simulink model "lin_model"  (R2014a)
settings: Solver=ode45  StartTime=0.0  StopTime=0.01  RelTol=1e-3
model workspace (MAT data in the model file):
  Ki = 12447149.4811
  Kd = -86.1936978403
  Kp = 336087.390249
settings Model: Creator=Deadok  LastModifiedBy=Mihail
settings DataIOCC: SignalLoggingSaveFormat=ModelDataLogs
settings OptimizationCC: ExpressionDepthLimit=2147483647
settings DebuggingCC: AlgebraicLoopMsg=none  UnderspecifiedInitializationDetection=Classic  SolverPrmCheckMsg=none  FcnCallInpInsideContextMsg=UseLocalSettings  UnconnectedInputMsg=none  UnconnectedOutputMsg=none  UnconnectedLineMsg=none  StateNameClashWarn=warning
settings GRTTargetCC: CombineOutputUpdateFcns=off  GRTInterface=on

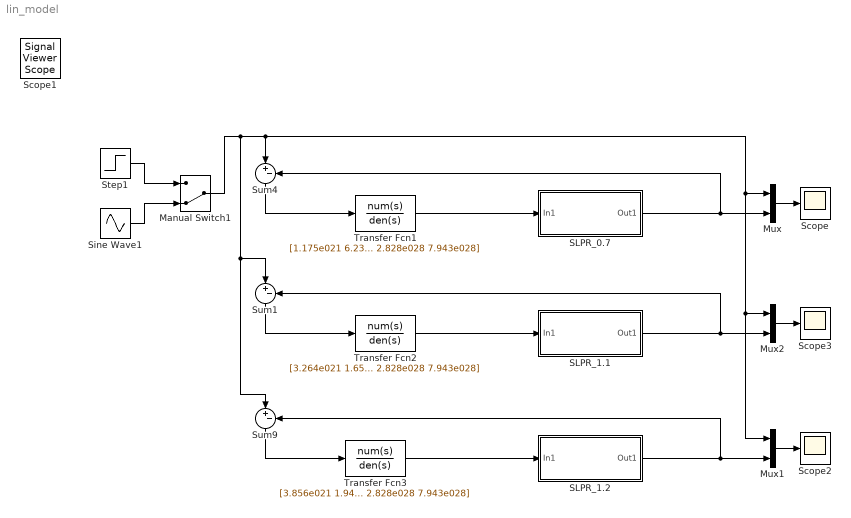
== system lin_model ==
  Manual Switch1 : ManualSwitch  CurrentSetting=0
  Mux : Mux  Inputs=2
  Mux1 : Mux  Inputs=2
  Mux2 : Mux  Inputs=2
  SLPR_0.7 : Subsystem
  SLPR_1.1 : Subsystem
  SLPR_1.2 : Subsystem
  Scope : Scope
      settings: TimeRange=16  YMin=1.832061068702288  YMax=5.832061068702288
  Scope2 : Scope
      settings: TimeRange=16  YMin=1.832061068702288  YMax=5.832061068702288
  Scope3 : Scope
      settings: TimeRange=16  YMin=1.832061068702288  YMax=5.832061068702288  SaveName=ScopeData2
  Sine Wave1 : Sin  Frequency=2000  SampleTime=0
  Step1 : Step  Time=0  SampleTime=0
  Sum1 : Sum  Inputs=|+-
  Sum4 : Sum  Inputs=|+-
  Sum9 : Sum  Inputs=|+-
  Transfer Fcn1 : TransferFcn  Numerator=[1.175e021 6.235e024 6.654e027 1.224e031 2.049e033 4.008e034 4.923e036 2.383e036]  Denominator=[1 1.539e006 8.565e011 2.152e017 2.439e022 1.001e027 2.828e028 7.943e028]
  Transfer Fcn2 : TransferFcn  Numerator=[3.264e021 1.656e025 1.052e028 1.263e031 2.055e033 4.055e034 4.923e036 2.383e036]  Denominator=[1 1.539e006 8.565e011 2.152e017 2.439e022 1.001e027 2.828e028 7.943e028]
  Transfer Fcn3 : TransferFcn  Numerator=[3.856e021 1.946e025 1.147e028 1.272e031 2.057e033 4.065e034 4.923e036 2.383e036]  Denominator=[1 1.539e006 8.565e011 2.152e017 2.439e022 1.001e027 2.828e028 7.943e028]
  Scope1 : SignalViewerScope  IOType=viewer  RefreshTime=0.035000
  wires:
  SLPR_0.7/1(Out1) -> Mux/2, Sum4/2
  Mux/1 -> Scope/1
  SLPR_1.2/1(Out1) -> Mux1/2, Sum9/2
  Sum9/1 -> Transfer Fcn3/1
  Mux1/1 -> Scope2/1
  SLPR_1.1/1(Out1) -> Sum1/2, Mux2/2
  Sine Wave1/1 -> Manual Switch1/2
  Step1/1 -> Manual Switch1/1
  Sum1/1 -> Transfer Fcn2/1
  Mux2/1 -> Scope3/1
  Manual Switch1/1 -> Sum1/1, Sum9/1, Sum4/1, Mux/1, Mux2/1, Mux1/1
  Sum4/1 -> Transfer Fcn1/1
  Transfer Fcn1/1 -> SLPR_0.7/1(In1)
  Transfer Fcn3/1 -> SLPR_1.2/1(In1)
  Transfer Fcn2/1 -> SLPR_1.1/1(In1)

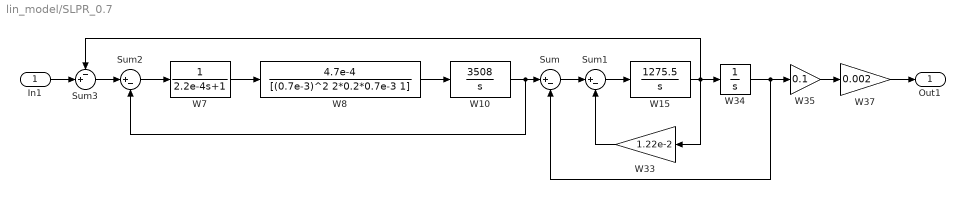
== system lin_model/SLPR_0.7 ==
  In1 : Inport
  Sum : Sum  Inputs=|+-
  Sum1 : Sum  Inputs=|+-
  Sum2 : Sum  Inputs=|+-
  Sum3 : Sum  Inputs=-+|
  W10 : TransferFcn  Numerator=[3508]  Denominator=[1 0]
  W15 : TransferFcn  Numerator=[1275.5]  Denominator=[1 0]
  W33 : Gain  Gain=1.22e-2
  W34 : Integrator
  W35 : Gain  Gain=0.1
  W37 : Gain  Gain=0.002
  W7 : TransferFcn  Denominator=[2.2e-4 1]
  W8 : TransferFcn  Numerator=[4.7e-4]  Denominator=[(0.7e-3)^2 2*0.2*0.7e-3 1]
  Out1 : Outport
  wires:
  W7/1 -> W8/1
  W8/1 -> W10/1
  W10/1 -> Sum2/2, Sum/1
  Sum/1 -> Sum1/1
  Sum1/1 -> W15/1
  W34/1 -> Sum/2, W35/1
  W33/1 -> Sum1/2
  Sum2/1 -> W7/1
  Sum3/1 -> Sum2/1
  W35/1 -> W37/1
  In1/1 -> Sum3/2
  W37/1 -> Out1/1
  W15/1 -> Sum3/1, W33/1, W34/1

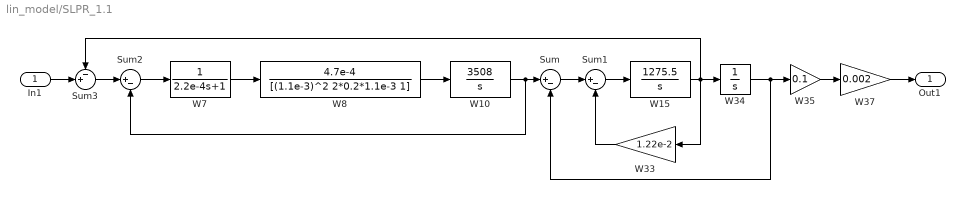
== system lin_model/SLPR_1.1 ==
  In1 : Inport
  Sum : Sum  Inputs=|+-
  Sum1 : Sum  Inputs=|+-
  Sum2 : Sum  Inputs=|+-
  Sum3 : Sum  Inputs=-+|
  W10 : TransferFcn  Numerator=[3508]  Denominator=[1 0]
  W15 : TransferFcn  Numerator=[1275.5]  Denominator=[1 0]
  W33 : Gain  Gain=1.22e-2
  W34 : Integrator
  W35 : Gain  Gain=0.1
  W37 : Gain  Gain=0.002
  W7 : TransferFcn  Denominator=[2.2e-4 1]
  W8 : TransferFcn  Numerator=[4.7e-4]  Denominator=[(1.1e-3)^2 2*0.2*1.1e-3 1]
  Out1 : Outport
  wires:
  W7/1 -> W8/1
  W8/1 -> W10/1
  W10/1 -> Sum2/2, Sum/1
  Sum/1 -> Sum1/1
  Sum1/1 -> W15/1
  W34/1 -> Sum/2, W35/1
  W33/1 -> Sum1/2
  Sum2/1 -> W7/1
  Sum3/1 -> Sum2/1
  W35/1 -> W37/1
  In1/1 -> Sum3/2
  W37/1 -> Out1/1
  W15/1 -> Sum3/1, W33/1, W34/1

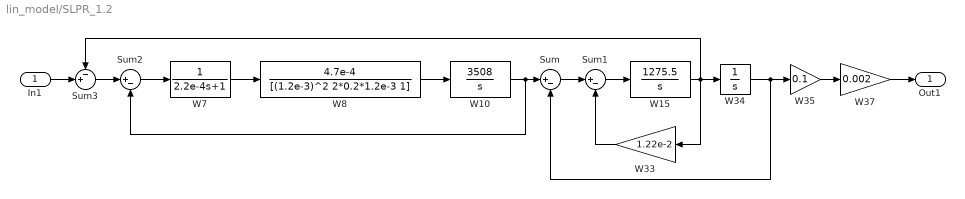
== system lin_model/SLPR_1.2 ==
  In1 : Inport
  Sum : Sum  Inputs=|+-
  Sum1 : Sum  Inputs=|+-
  Sum2 : Sum  Inputs=|+-
  Sum3 : Sum  Inputs=-+|
  W10 : TransferFcn  Numerator=[3508]  Denominator=[1 0]
  W15 : TransferFcn  Numerator=[1275.5]  Denominator=[1 0]
  W33 : Gain  Gain=1.22e-2
  W34 : Integrator
  W35 : Gain  Gain=0.1
  W37 : Gain  Gain=0.002
  W7 : TransferFcn  Denominator=[2.2e-4 1]
  W8 : TransferFcn  Numerator=[4.7e-4]  Denominator=[(1.2e-3)^2 2*0.2*1.2e-3 1]
  Out1 : Outport
  wires:
  W7/1 -> W8/1
  W8/1 -> W10/1
  W10/1 -> Sum2/2, Sum/1
  Sum/1 -> Sum1/1
  Sum1/1 -> W15/1
  W34/1 -> Sum/2, W35/1
  W33/1 -> Sum1/2
  Sum2/1 -> W7/1
  Sum3/1 -> Sum2/1
  W35/1 -> W37/1
  In1/1 -> Sum3/2
  W37/1 -> Out1/1
  W15/1 -> Sum3/1, W33/1, W34/1
